simulink model "zweipunktregler"  (R2016a)
settings: Solver=FixedStepAuto  StartTime=0.0  StopTime=800  RelTol=1e-3
settings Model: Creator=Hello Cao  LastModifiedBy=HaloCao
settings DataIOCC: LimitDataPoints=on  SaveFormat=Array
settings DebuggingCC: MaxConsecutiveZCsMsg=none
settings HardwareCC: ProdLargestAtomicFloat=None  ProdIntDivRoundTo=Undefined  ProdEndianess=Unspecified  ProdWordSize=32  ProdHWDeviceType=Generic->64-bit Embedded Processor (LLP64)  TargetBitPerPointer=64  TargetLongLongMode=on  TargetIntDivRoundTo=Zero  TargetEndianess=LittleEndian  TargetWordSize=64  TargetHWDeviceType=MATLAB Host  ProdEqTarget=off
settings ModelReferenceCC: PropagateSignalLabelsOutOfModel=off
settings ConfigComp: CovModelRefEnable=Off  CovSFcnEnable=off

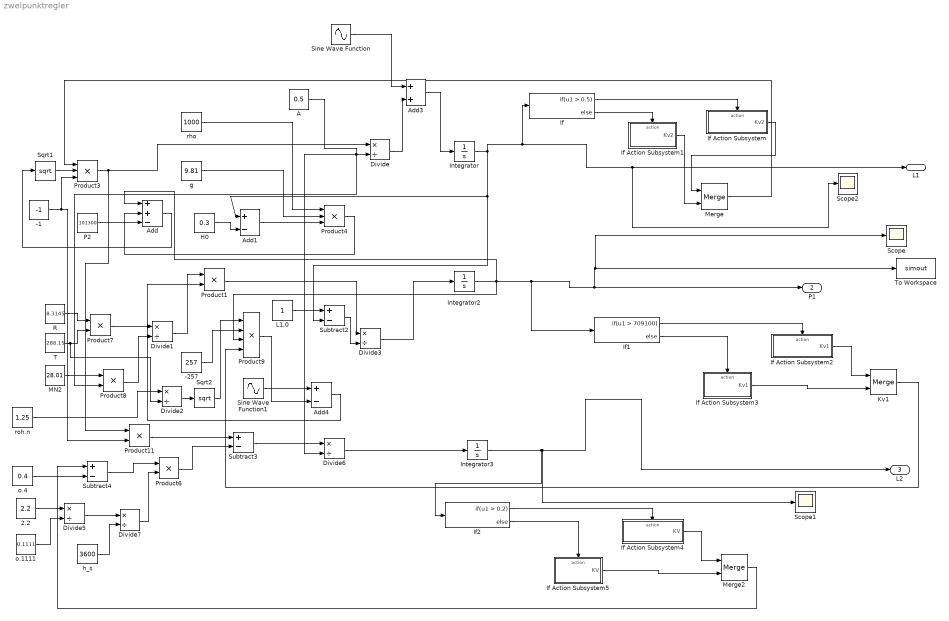
== system zweipunktregler ==
  -1 : Constant  Value=-1
  -257 : Constant  Value=257
  2.2 : Constant  Value=2.2
  A : Constant  Value=0.5
  Add : Sum  Inputs=++-
  Add1 : Sum  Inputs=+-
  Add3 : Sum
  Add4 : Sum  Inputs=+-
  Divide{,1..3,5..7} (7 alike) : Product  Inputs=*/
  H0 : Constant  Value=0.3
  If : If  IfExpression=u1 > 0.5
  If Action Subsystem : Subsystem  TreatAsAtomicUnit=on
  If Action Subsystem1 : Subsystem  TreatAsAtomicUnit=on
  If Action Subsystem2 : Subsystem  TreatAsAtomicUnit=on
  If Action Subsystem3 : Subsystem  TreatAsAtomicUnit=on
  If Action Subsystem4 : Subsystem  TreatAsAtomicUnit=on
  If Action Subsystem5 : Subsystem  TreatAsAtomicUnit=on
  If1 : If  IfExpression=u1 > 709100
  If2 : If  IfExpression=u1 > 0.2
  Integrator : Integrator
  Integrator2 : Integrator  InitialCondition=3212009
  Integrator3 : Integrator
  Kv1 : Merge
  L1,0 : Constant
  MN2 : Constant  Value=28.01
  Merge : Merge
  Merge2 : Merge
  P2 : Constant  Value=101300
  Product{1,6..8,11} (5 alike) : Product
  Product3 : Product  Inputs=3
  Product4 : Product  Inputs=3
  Product9 : Product  Inputs=4
  R : Constant  Value=8.3145
  Scope : Scope
  Scope1 : Scope
  Scope2 : Scope
  Sine Wave Function : Sin  Amplitude=0.0001  Bias=0.001  SampleTime=0
  Sine Wave Function1 : Sin  Bias=10  SampleTime=0
  Sqrt1 : Sqrt  SaturateOnIntegerOverflow=on
  Sqrt2 : Sqrt  SaturateOnIntegerOverflow=on
  Subtract2 : Sum  Inputs=+-
  Subtract3 : Sum  Inputs=+-
  Subtract4 : Sum  Inputs=+-
  T : Constant  Value=288.15
  To Workspace : ToWorkspace  VariableName=simout  SaveFormat=Timeseries  SampleTime=-1
  g : Constant  Value=9.81
  h_s : Constant  Value=3600
  o.1111 : Constant  Value=0.1111
  o.4 : Constant  Value=0.4
  rho : Constant  Value=1000
  roh.n : Constant  Value=1.25
  L1 : Outport
  P1 : Outport  Port=2
  L2 : Outport  Port=3
  wires:
  Integrator/1 -> If/1, Scope2/1, L1/1, Subtract2/2, Add1/1
  Sqrt1/1 -> Product3/2
  Add/1 -> Sqrt1/1
  H0/1 -> Add1/2
  rho/1 -> Product4/1
  g/1 -> Product4/2
  Add1/1 -> Product4/3
  Product4/1 -> Add/2
  P2/1 -> Add/3
  A/1 -> Divide6/2, Product8/2, Divide/2
  Divide/1 -> Add3/2
  R/1 -> Product7/1
  T/1 -> Divide2/2, Product7/2
  Product7/1 -> Divide1/1
  MN2/1 -> Product8/1
  Product8/1 -> Divide1/2
  -257/1 -> Product9/2
  Divide2/1 -> Sqrt2/1
  Sqrt2/1 -> Product9/1
  L1,0/1 -> Subtract2/1
  Subtract2/1 -> Divide3/2
  Divide3/1 -> Integrator2/1
  -1/1 -> Product11/2, Product3/3
  Product3/1 -> Product11/1, Divide/1
  Product11/1 -> Subtract3/1
  Product6/1 -> Subtract3/2
  Subtract4/1 -> Product6/1
  o.4/1 -> Subtract4/2
  2.2/1 -> Divide5/1
  o.1111/1 -> Divide5/2
  Subtract3/1 -> Divide6/1
  Divide6/1 -> Integrator3/1
  If/1 -> If Action Subsystem/Action
  If/2 -> If Action Subsystem1/Action
  If Action Subsystem/1(Kv2) -> Merge/1
  If Action Subsystem1/1(Kv2) -> Merge/2
  Merge/1 -> Product3/1
  Integrator2/1 -> Add/1, If1/1, Scope/1, To Workspace/1, P1/1, Product9/3
  If Action Subsystem2/1(Kv1) -> Kv1/1
  If Action Subsystem3/1(Kv1) -> Kv1/2
  Kv1/1 -> Product9/4
  If1/2 -> If Action Subsystem3/Action
  If1/1 -> If Action Subsystem2/Action
  Integrator3/1 -> Scope1/1, L2/1, If2/1
  If Action Subsystem4/1(KV) -> Merge2/1
  If Action Subsystem5/1(KV) -> Merge2/2
  Merge2/1 -> Subtract4/1
  If2/1 -> If Action Subsystem4/Action
  If2/2 -> If Action Subsystem5/Action
  Sine Wave Function/1 -> Add3/1
  Add3/1 -> Integrator/1
  Sine Wave Function1/1 -> Add4/1
  roh.n/1 -> Divide2/1
  Product9/1 -> Add4/2
  Add4/1 -> Product1/2
  Divide1/1 -> Product1/1
  Product1/1 -> Divide3/1
  Divide5/1 -> Divide7/1
  Divide7/1 -> Product6/2
  h_s/1 -> Divide7/2

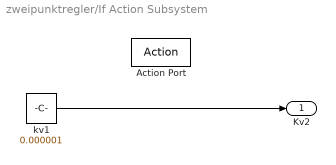
== system zweipunktregler/If Action Subsystem ==
  Action Port : ActionPort  ActionType=then
  kv1 : Constant  Value=0.000001
  Kv2 : Outport
  wires:
  kv1/1 -> Kv2/1

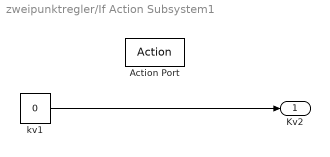
== system zweipunktregler/If Action Subsystem1 ==
  Action Port : ActionPort  ActionType=else
  kv1 : Constant  Value=0
  Kv2 : Outport
  wires:
  kv1/1 -> Kv2/1

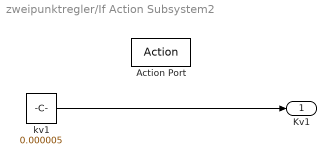
== system zweipunktregler/If Action Subsystem2 ==
  Action Port : ActionPort  ActionType=then
  kv1 : Constant  Value=0.000005  VectorParams1D=off
  Kv1 : Outport
  wires:
  kv1/1 -> Kv1/1

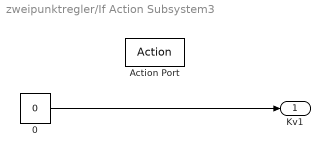
== system zweipunktregler/If Action Subsystem3 ==
  Action Port : ActionPort  ActionType=else
  0 : Constant  Value=0
  Kv1 : Outport
  wires:
  0/1 -> Kv1/1

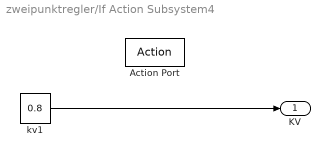
== system zweipunktregler/If Action Subsystem4 ==
  Action Port : ActionPort  PropagateVarSize=During execution  ActionType=then
  kv1 : Constant  Value=0.8
  KV : Outport
  wires:
  kv1/1 -> KV/1

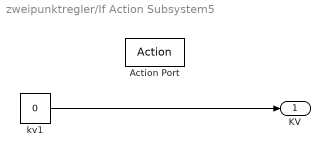
== system zweipunktregler/If Action Subsystem5 ==
  Action Port : ActionPort  ActionType=else
  kv1 : Constant  Value=0
  KV : Outport
  wires:
  kv1/1 -> KV/1
